simulink model "sim1_unlinear_model_with_LQR"  (R2023b)
settings: Solver=FixedStepAuto  StartTime=0.0  StopTime=20  FixedStep=0.001  MaxStep=0.01  RelTol=1e-3
values from neighbouring files (symbols this model uses):
  K = lqr(A, B, Q, R)    [s2_mathematical_model.m]
  x0 = [x_v_0; v_v_x_0; theta_v_y_0; D_theta_v_y_0; psi_v_z_0; D_psi_v_z_0]    [s2_mathematical_model.m]
undefined symbols (not defined in the file or in its folder): Params, sigbuilder_block
settings Model: Creator=tutaj  LastModifiedBy=wojte
settings OptimizationCC: ReuseModelBlockBuffer=off

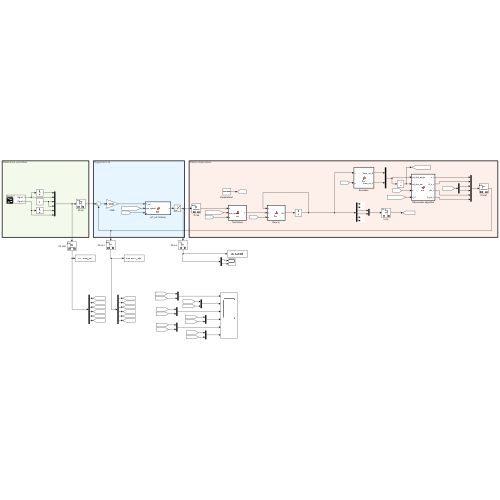
[thumbnail: Simulink's stored preview of the top-level diagram]
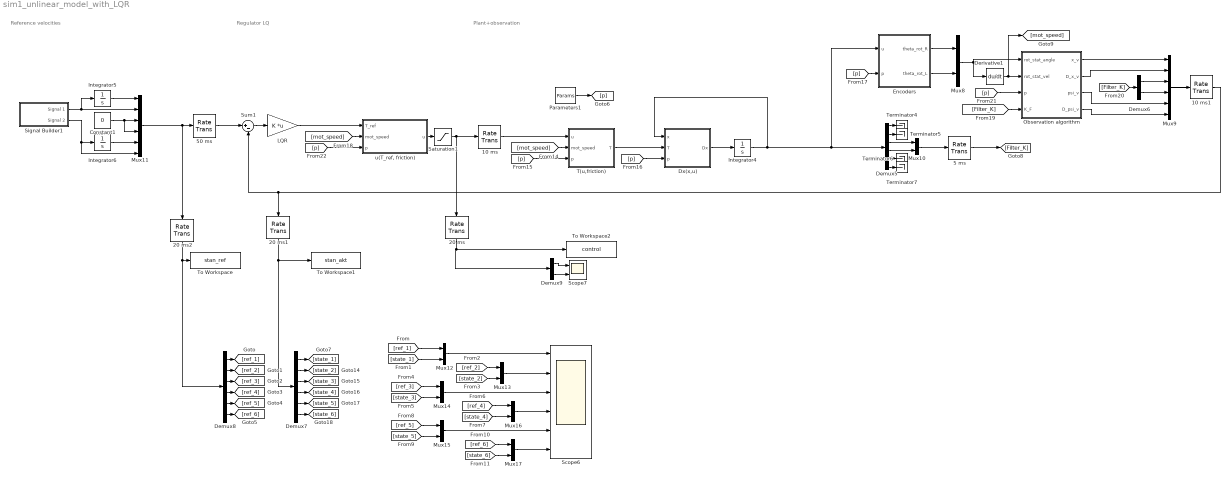
== system sim1_unlinear_model_with_LQR ==
  note: Regulator LQ
  note: Plant+observation
  note: Reference velocities
  10 ms : RateTransition  OutPortSampleTime=0.01
  10 ms1 : RateTransition  OutPortSampleTime=0.01
  20 ms : RateTransition  OutPortSampleTime=0.02
  20 ms1 : RateTransition  OutPortSampleTime=0.02
  20 ms2 : RateTransition  OutPortSampleTime=0.02
  5 ms : RateTransition  OutPortSampleTime=0.005
  50 ms : RateTransition  OutPortSampleTime=0.05
  Constant1 : Constant  Value=0
  Demux5 : Demux  Outputs=6
  Demux6 : Demux  Outputs=2
  Demux7 : Demux  Outputs=6
  Demux8 : Demux  Outputs=6
  Demux9 : Demux  Outputs=2
  Derivative1 : Derivative
  Dx(x,u) : MATLAB Function  TreatAsAtomicUnit=on
  Encoders : MATLAB Function  TreatAsAtomicUnit=on
  Integrator4 : Integrator  InitialCondition=x0
  Integrator5 : Integrator
  Integrator6 : Integrator
  "LQR " : Gain  Gain=K  Multiplication=Matrix(K*u) (u vector)
  Mux{8,10,12..17} (8 alike) : Mux  Inputs=2
  Mux11 : Mux  Inputs=6
  Mux9 : Mux  Inputs=6
  Observation algorithm : MATLAB Function  TreatAsAtomicUnit=on
  Parameters1 : Constant  Value=Params
  Saturation1 : Saturate  UpperLimit=12  LowerLimit=-12
  Scope6 : Scope  NumInputPorts=6
  Scope7 : Scope  NumInputPorts=2
  Signal Builder1 : Subsystem  Tag=STV Subsys  LoadFcn=sigbuilder_block('load');  StartFcn=sigbuilder_block('start');  StopFcn=sigbuilder_block('stop');  ClipboardFcn=sigbuilder_block('clipboard');  mask(Sigbuilder block){tuvar=[0:10]}
      mask help: Simulink:masks:SigbuilderBlock_MD
      mask init:
      | if ~strcmp(get_param(bdroot(gcbh),'SimulationStatus'),'stopped') tuvar = sigbuilder_block('maskInit'); end
      settings: CopyFcn=sigbuilder_block('copy');  DeleteFcn=sigbuilder_block('delete');  ModelCloseFcn=sigbuilder_block('modelClose');  PreSaveFcn=sigbuilder_block('preSave');  PauseFcn=sigbuilder_block('pause');  ContinueFcn=sigbuilder_block('continue');  NameChangeFcn=sigbuilder_block('namechange');  OpenFcn=sigbuilder_block('open',[391.2 154.2 550.8 399.6 ]);  CloseFcn=sigbuilder_block('close');
      mask Display: plot(0, 0, 100, 100,[2, 2, 32, 32, 2], [68, 8, 8, 68, 68],[32, 2], [38, 38], [32, 19, 2],[53, 60, 44], [32, 17, 17, 2],[16, 16, 31, 31]);txt = getActiveGroup(gcbh);text(2, 100, txt,'verticalAlignment', 'top');
  Sum1 : Sum  Inputs=|+-
  T(u,friction) : MATLAB Function  TreatAsAtomicUnit=on
  Terminator{4..7} (4 alike) : Terminator
  To Workspace : ToWorkspace  VariableName=stan_ref  SampleTime=-1
  To Workspace1 : ToWorkspace  VariableName=stan_akt  SampleTime=-1
  To Workspace2 : ToWorkspace  VariableName=control  SampleTime=-1
  "u(T_ref, friction)" : MATLAB Function  TreatAsAtomicUnit=on
  wires:
  [p] -> Dx(x,u)/3(p)
  T(u,friction)/1(T) -> Dx(x,u)/2(T)
  Demux5/1 -> Terminator4/1
  [mot_speed] -> T(u,friction)/2(mot_speed)
  Derivative1/1 -> [mot_speed], Observation algorithm/2(rot_stat_vel)
  Encoders/1(theta_rot_R) -> Mux8/1
  Demux5/3 -> Mux10/1
  Demux6/2 -> Mux9/4
  Mux10/1 -> 5 ms/1
  Demux5/5 -> Terminator6/1
  Observation algorithm/4(D_psi_v) -> Mux9/6
  Demux6/1 -> Mux9/3
  Demux5/2 -> Terminator5/1
  Observation algorithm/2(D_x_v) -> Mux9/2
  [p] -> Encoders/2(p)
  Observation algorithm/3(psi_v) -> Mux9/5
  Dx(x,u)/1(Dx) -> Integrator4/1
  [p] -> T(u,friction)/3(p)
  Parameters1/1 -> [p]
  Demux5/6 -> Terminator7/1
  Observation algorithm/1(x_v) -> Mux9/1
  Mux8/1 -> Derivative1/1, Observation algorithm/1(rot_stat_angle)
  [Filter_K] -> Demux6/1
  [p] -> Observation algorithm/3(p)
  Encoders/2(theta_rot_L) -> Mux8/2
  Demux5/4 -> Mux10/2
  Integrator4/1 -> Dx(x,u)/1(x), Encoders/1(u), Demux5/1
  [Filter_K] -> Observation algorithm/4(K_F)
  "u(T_ref, friction)"/1(u) -> Saturation1/1
  [mot_speed] -> "u(T_ref, friction)"/2(mot_speed)
  [p] -> "u(T_ref, friction)"/3(p)
  "LQR "/1 -> "u(T_ref, friction)"/1(T_ref)
  Sum1/1 -> "LQR "/1
  Mux9/1 -> 10 ms1/1
  Saturation1/1 -> 20 ms/1, 10 ms/1
  Demux9/2 -> Scope7/2
  Demux9/1 -> Scope7/1
  50 ms/1 -> Sum1/1
  10 ms/1 -> T(u,friction)/1(u)
  5 ms/1 -> [Filter_K]
  10 ms1/1 -> Sum1/2, 20 ms1/1
  20 ms/1 -> Demux9/1, To Workspace2/1
  20 ms1/1 -> Demux7/1, To Workspace1/1
  20 ms2/1 -> Demux8/1, To Workspace/1
  Integrator5/1 -> Mux11/1
  Integrator6/1 -> Mux11/5
  Constant1/1 -> Mux11/3, Mux11/4
  Signal Builder1/1(Signal 1) -> Integrator5/1, Mux11/2
  Signal Builder1/2(Signal 2) -> Mux11/6, Integrator6/1
  Mux11/1 -> 20 ms2/1, 50 ms/1
  Demux8/1 -> [ref_1]
  Demux8/2 -> [ref_2]
  Demux8/3 -> [ref_3]
  Demux8/4 -> [ref_4]
  Demux8/5 -> [ref_5]
  Demux8/6 -> [ref_6]
  Demux7/1 -> [state_1]
  Demux7/2 -> [state_2]
  Demux7/3 -> [state_3]
  Demux7/4 -> [state_4]
  Demux7/5 -> [state_5]
  Demux7/6 -> [state_6]
  Mux12/1 -> Scope6/1
  [ref_1] -> Mux12/1
  [state_1] -> Mux12/2
  Mux13/1 -> Scope6/2
  [ref_2] -> Mux13/1
  [state_2] -> Mux13/2
  [ref_3] -> Mux14/1
  [state_3] -> Mux14/2
  [ref_4] -> Mux16/1
  [state_4] -> Mux16/2
  Mux16/1 -> Scope6/4
  Mux14/1 -> Scope6/3
  [state_6] -> Mux17/2
  [ref_6] -> Mux17/1
  Mux17/1 -> Scope6/6
  [ref_5] -> Mux15/1
  [state_5] -> Mux15/2
  Mux15/1 -> Scope6/5

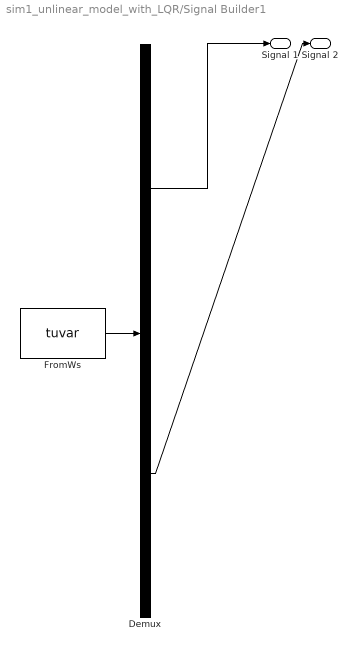
== system sim1_unlinear_model_with_LQR/Signal Builder1 ==
  Demux : Demux  Tag=STV Demux  Outputs=2
      settings: DisplayOption=none
  FromWs : FromWorkspace  Tag=STV FromWs  VariableName=tuvar
      SigBuilderData=|
      | common.afterFinalStr = 'Extrapolate'
      | common.sampleTime = 0
      | dataSet.timeRange = [0 20]
      | dataSet.name = 'Group 1'
      | sbobj.Groups.Name = 'Group 1'
      | sbobj.Groups.Signals(1).Name = 'Signal 1'
      | sbobj.Groups.Signals(1).XData = [0 10 11 12 13 20]
      | sbobj.Groups.Signals(1).YData = [0 0 0.2 0.2 0 0]
      | sbobj.Groups.Signals(2).Name = 'Signal 2'
      | sbobj.Groups.Signals(2).XData = [0 5 6 7 8 20]
      | sbobj.Groups.Signals(2).YData = [0 0 0.1 0.1 0 0]
      | sbobj.Groups.TimeRange = [0 20]
  Signal 1 : Outport  Tag=STV Outport
  Signal 2 : Outport  Tag=STV Outport  Port=2
  wires:
  Demux/1 -> Signal 1/1
  FromWs/1 -> Demux/1
  Demux/2 -> Signal 2/1

== matlab function sim1_unlinear_model_with_LQR/Observation algorithm ==
  data: rot_stat_angle input; rot_stat_vel input; x_v output; D_x_v output; psi_v output; p input; K_F input; D_psi_v output
function [x_v, D_x_v, psi_v, D_psi_v] = fcn(rot_stat_angle, rot_stat_vel, p, K_F)

D = p(3);
r = p(4);

theta_rot_R = rot_stat_angle(1);
theta_rot_L = rot_stat_angle(2);
D_theta_rot_R = rot_stat_vel(1);
D_theta_rot_L = rot_stat_vel(2);
theta_v_y = K_F(1);
D_theta_v_y = K_F(2);


x_v = ((theta_rot_R + theta_rot_L)/2 + theta_v_y)*r;
D_x_v = ((D_theta_rot_R + D_theta_rot_L)/2 + D_theta_v_y)*r;
psi_v = (theta_rot_R - theta_rot_L)*r/D;
D_psi_v = (D_theta_rot_R - D_theta_rot_L)*r/D;

== matlab function sim1_unlinear_model_with_LQR/T(u,friction) ==
  data: u input; T output; mot_speed input; p input
function T = fcn(u, mot_speed, p)

T = zeros(2,1);
u_R = u(1);
u_L = u(2);

omega_mot_R = mot_speed(1);
omega_mot_L = mot_speed(2);

b_Coul_R = p(12);
b_visc_R = p(13);
b_Coul_L = p(14);
b_visc_L = p(15);
R = p(16);
k_e = p(17);
k_m = p(18);
% L_m = Params(19); (induktance omitted)

T_R= k_m*u_R/R + (-k_m*k_e/R - b_visc_R)*omega_mot_R - b_Coul_R*sign(omega_mot_R);
T_L= k_m*u_L/R + (-k_m*k_e/R - b_visc_L)*omega_mot_L - b_Coul_L*sign(omega_mot_L);
T_theta_t = T_R + T_L;
T_psi_t = T_R - T_L;

T(1) = T_theta_t;
T(2) = T_psi_t;

== matlab function sim1_unlinear_model_with_LQR/Dx(x,u) ==
  data: x input; T input; Dx output; p input
function Dx = fcn(x,T,p)

I_v_axle_x_t = x(1);
v_axle_x_t = x(2);
theta_v_y_t = x(3);
D_theta_v_y_t = x(4);
psi_z_t = x(5);
D_psi_v_z_t = x(6);

T_theta_t = T(1);
T_psi_t = T(2);

g = p(1);
L = p(2);
D = p(3);
r = p(4);
J_v_x = p(5);
J_v_y = p(6);
J_v_z = p(7);
m_v = p(8);
J_w_xz = p(9);
J_w_y = p(10);
m_w = p(11);

Dx = [
    v_axle_x_t
    (r*(2*J_v_y*T_theta_t + 2*L^2*T_theta_t*m_v + 2*L*T_theta_t*m_v*r*cos(theta_v_y_t) + 2*D_theta_v_y_t^2*L^3*m_v^2*r*sin(theta_v_y_t) - 2*D_psi_v_z_t^2*L^3*m_v^2*r*cos(theta_v_y_t)^2*sin(theta_v_y_t) + 2*D_theta_v_y_t^2*J_v_y*L*m_v*r*sin(theta_v_y_t) - 2*L^2*g*m_v^2*r*cos(theta_v_y_t)*sin(theta_v_y_t) - 2*D_psi_v_z_t^2*J_v_x*L*m_v*r*cos(theta_v_y_t)^2*sin(theta_v_y_t) + 2*D_psi_v_z_t^2*J_v_z*L*m_v*r*cos(theta_v_y_t)^2*sin(theta_v_y_t)))/(2*(2*J_v_y*J_w_y + L^2*m_v^2*r^2 + 2*J_w_y*L^2*m_v + J_v_y*m_v*r^2 + 2*J_v_y*m_w*r^2 + 2*L^2*m_v*m_w*r^2 - L^2*m_v^2*r^2*cos(theta_v_y_t)^2))
    D_theta_v_y_t
    (2*D_psi_v_z_t^2*J_v_x*J_w_y*sin(2*theta_v_y_t) - 2*T_theta_t*m_v*r^2 - 4*T_theta_t*m_w*r^2 - 4*J_w_y*T_theta_t - 2*D_psi_v_z_t^2*J_v_z*J_w_y*sin(2*theta_v_y_t) + D_psi_v_z_t^2*L^2*m_v^2*r^2*sin(2*theta_v_y_t) - D_theta_v_y_t^2*L^2*m_v^2*r^2*sin(2*theta_v_y_t) + 2*L*g*m_v^2*r^2*sin(theta_v_y_t) + 2*D_psi_v_z_t^2*J_w_y*L^2*m_v*sin(2*theta_v_y_t) + 4*J_w_y*L*g*m_v*sin(theta_v_y_t) - 2*L*T_theta_t*m_v*r*cos(theta_v_y_t) + D_psi_v_z_t^2*J_v_x*m_v*r^2*sin(2*theta_v_y_t) - D_psi_v_z_t^2*J_v_z*m_v*r^2*sin(2*theta_v_y_t) + 2*D_psi_v_z_t^2*J_v_x*m_w*r^2*sin(2*theta_v_y_t) - 2*D_psi_v_z_t^2*J_v_z*m_w*r^2*sin(2*theta_v_y_t) + 2*D_psi_v_z_t^2*L^2*m_v*m_w*r^2*sin(2*theta_v_y_t) + 4*L*g*m_v*m_w*r^2*sin(theta_v_y_t))/(4*J_v_y*J_w_y + L^2*m_v^2*r^2 + 4*J_w_y*L^2*m_v + 2*J_v_y*m_v*r^2 + 4*J_v_y*m_w*r^2 + 4*L^2*m_v*m_w*r^2 - L^2*m_v^2*r^2*cos(2*theta_v_y_t))
    D_psi_v_z_t
    (r*(- 2*D_psi_v_z_t*D_theta_v_y_t*m_v*r*sin(2*theta_v_y_t)*L^2 + T_psi_t*D - 2*D_psi_v_z_t*D_theta_v_y_t*J_v_x*r*sin(2*theta_v_y_t) + 2*D_psi_v_z_t*D_theta_v_y_t*J_v_z*r*sin(2*theta_v_y_t)))/(D^2*J_w_y + 2*J_v_x*r^2 + 4*J_w_xz*r^2 + D^2*m_w*r^2 + 2*L^2*m_v*r^2 - 2*J_v_x*r^2*cos(theta_v_y_t)^2 + 2*J_v_z*r^2*cos(theta_v_y_t)^2 - 2*L^2*m_v*r^2*cos(theta_v_y_t)^2)
    ];

== matlab function sim1_unlinear_model_with_LQR/Encoders ==
  data: u input; theta_rot_R output; theta_rot_L output; p input
function [theta_rot_R,theta_rot_L] = fcn(u, p)

D = p(3);
r = p(4);

x_v = u(1);
theta_v_y = u(3);
psi_v = u(5);

theta_rot_R = (2*x_v + D*psi_v - 2*r*theta_v_y)/(2*r);
theta_rot_L = -(D*psi_v - 2*x_v + 2*r*theta_v_y)/(2*r);

== matlab function sim1_unlinear_model_with_LQR/u(T_ref, friction) ==
  data: T_ref input; u output; mot_speed input; p input
function u = fcn(T_ref, mot_speed, p)
u = zeros(2, 1);

T_theta_t = T_ref(1);
T_psi_t = T_ref(2);

T_R = (T_theta_t + T_psi_t)/2;
T_L = (T_theta_t - T_psi_t)/2;

omega_mot_R = mot_speed(1);
omega_mot_L = mot_speed(2);

b_Coul_R = p(12);
b_visc_R = p(13);
b_Coul_L = p(14);
b_visc_L = p(15);

R = p(16);
k_e = p(17);
k_m = p(18);
% L_m = Params(19); (induktance omitted) 

u(1)= R/k_m*(T_R - (-k_m*k_e/R - b_visc_R)*omega_mot_R + b_Coul_R*sign(omega_mot_R));
u(2)= R/k_m*(T_L - (-k_m*k_e/R - b_visc_L)*omega_mot_L + b_Coul_L*sign(omega_mot_L));
